simulink model "tesdoang"  (R2024a)
settings: Solver=FixedStepAuto  StartTime=0.0  StopTime=10  FixedStep=1e-5  RelTol=1e-3
values from neighbouring files (symbols this model uses):
  C_inv = (r*(Pinv/3)*al*(-be+al-1))/(100*Vac_l_rms*Vin_inv*wn*(al-be))    [main_v2gg2v.m]    (also in script.m = 0.00198943678865)
  C_mppt = 20*(Iout_mppt*D_mppt)/(deltaV*fs_mppt)    (= 0.0948148148148)    [main_v2gg2v.m]    (also in script.m)
  cap_bat = 2000    [main_v2gg2v.m]    (also in script.m)
  Cbat_buck = deltaI_bat/(8*fs_bat*deltaV_bat)    (= 0.00133333333333)    [main_v2gg2v.m]    (also in script.m)
  Cdc = 30e-3    (= 0.03)    [main_v2gg2v.m]    (also in script.m)
  Cdc_boost = 50*Cbat_buck    (= 0.0666666666667)    [main_v2gg2v.m]    (also in script.m)
  D_g1 = 5    [script.m]
  D_g2 = 5    [script.m]
  Elf_g1 = 1.06    [script.m]
  Elf_g2 = 1.15    [script.m]
  fg = 50    [main_v2gg2v.m]    (also in script.m)
  H_g1 = 4    [script.m]
  H_g2 = 1.8    [script.m]
  L_bat = (Vbat*(Vdc_link-Vbat))/(deltaI_bat*fs_bat*Vdc_link)    (= 0.001875)    [main_v2gg2v.m]    (also in script.m)
  L_mppt = 1*(Vpv*D_mppt)/(deltaI*fs_mppt)    (= 0.000161333333333)    [main_v2gg2v.m]    (also in script.m)
  Lmin_inv = (100*Vac_l_rms*Vin_inv*(al-be))/(wn*r*(Pinv/3)*(-be+al-1))    [main_v2gg2v.m]    (also in script.m = 0.000611154981473)
  pairPoles_g1 = 2    [script.m]
  pairPoles_g2 = 3    [script.m]
  Pinv = 2e6    (= 2000000)    [main_v2gg2v.m]    (also in script.m)
  Pmlf_g1 = 0.84    [script.m]
  Pmlf_g2 = 0.82    [script.m]
  R_g1 = 0.015    [script.m]
  R_g2 = 0.02    [script.m]
  Rdroop_g1 = 0.05    [script.m]
  Rdroop_g2 = 0.06    [script.m]
  RL_mppt_dummy = Vdc_link^2/Ppv    (= 1.125)    [main_v2gg2v.m]    (also in script.m)
  Sbase = 1e6    (= 1000000)    [main_v2gg2v.m]    (also in script.m)
  Snom_g1 = 7e6    (= 7000000)    [script.m]
  Snom_g2 = 5e6    (= 5000000)    [script.m]
  Tg_g1 = 0.4    [script.m]
  Tg_g2 = 0.25    [script.m]
  Vac_grid = Vbase    (= 345000)    [script.m]
  Vac_inv = 800    [main_v2gg2v.m]    (also in script.m)
  Vbat = 750    [main_v2gg2v.m]    (also in script.m)
  X_g1 = 0.3    [script.m]
  X_g2 = 0.35    [script.m]
  Xline_12 = 7/6    (= 1.16666666667)    [script.m]
  Xline_13 = 8/6    (= 1.33333333333)    [script.m]
  Xline_23 = 4/6    (= 0.666666666667)    [script.m]
  Zbase = Vbase^2/Sbase    (= 119025)    [main_v2gg2v.m]    (also in script.m)
undefined symbols (not defined in the file or in its folder): A, Acid, B, C, D1, Delta, DiscIntNeverNeededParam, K_lqr, L_kal, Lead
libraries: spsGroundLib x14, eeGeneralControl x10, spsSeriesRLCBranchLib x9, simulink x7, spsThreePhaseVIMeasurementLib x6, slpidlib x6, spsThreePhaseSeriesRLCBranchLib x6, spsCurrentMeasurementLib x5, spsBatteryLib x3, spsVoltageMeasurementLib x3, spsRMSLib x3, spsThreePhaseParallelRLCLoadLib x3
(part 1 of 2)
settings Model: SimulationMode=accelerator  Creator=hp  LastModifiedBy=hp
settings DebuggingCC: AlgebraicLoopMsg=error  ArtificialAlgebraicLoopMsg=error  BlockPriorityViolationMsg=error  SolverPrmCheckMsg=warning  StateNameClashWarn=warning  OperatingPointInterfaceChecksumMismatchMsg=error
settings HardwareCC: ProdHWDeviceType=AMD->x86-64 (Windows64)
settings DiagnosticsConfigSet: SimMechanicsInvalidVisualProperty=error  SimMechanicsCrossSectionNullEdge=error  SimMechanicsUnconnectedFramePorts=error  SimMechanicsUnconnectedGeometryPorts=error  SimMechanicsRedundantBlock=error  SimMechanicsConflictingReferenceFrames=error  SimMechanicsUnsatisfiedHighPriorityTargets=error

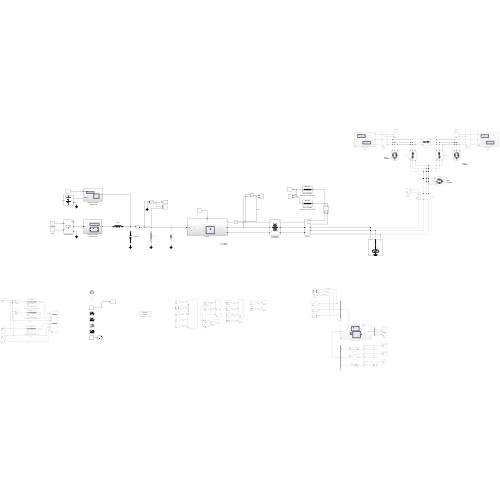
[thumbnail: Simulink's stored preview of the top-level diagram]
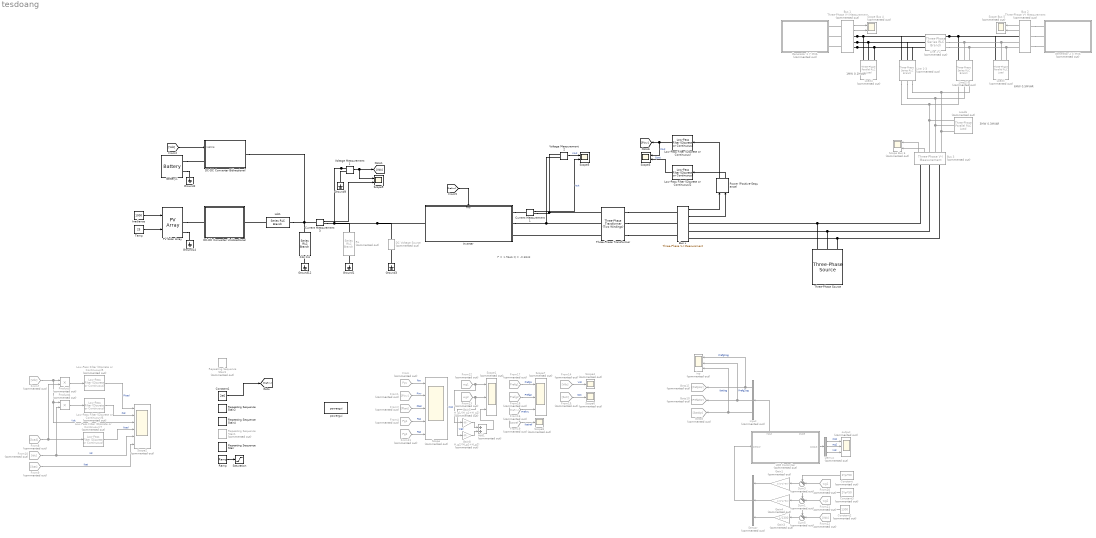
== system tesdoang ==
  note: P = 1.96e6
      | Q = -0.6843
  note: 6MW
      | 0.5MVAR
  note: 3MW
      | 0.3MVAR
  note: 1MW
      | 0.1MVAR
  Add1 : Sum  Commented=on
  Battery1 : spsBatteryLib/Battery  BatType=Lead-Acid  ShowTempParam=off  ThermalPreset="12.8V  40Ah  (LiFeMgPO4)"  ShowAgeParam=off  NomV=Vbat  NomQ=cap_bat  SOC=50  Batt_Tr=2  PresetModel=off  MaxQ=cap_bat  MinV=0.8*Vbat  FullV=1.1*Vbat  Dis_rate=Inom_bat  R=0.002  Normal_OP=0.9*cap_bat  expZone="[780   20]"  current=[250 500 750 1000]  Units=Ampere-hour  Tci=20  NomT=20  T2=-30  MaxQ2=4.8  FullV2=7.1  Normal_OP2=5.655  expZone2="[6.58           1]"  Rca=0.6  ti=2000  Dp=0  Neq0=0  Tsim=1e6  Ta1=25  Qeol=5.4*0.9  Reol=0.013333*1.2  Char_age=[2.3478, 3]  Dis_age=[2.3478, 10]  N1=1500  N2=10500  N3=1000  N4=1400  Ta2=45  N5=950
  Bus 1 : spsThreePhaseVIMeasurementLib/Three-Phase V-I Measurement  Commented=on  VoltageMeasurement=phase-to-phase  SetLabelV=off  LabelV=Vabc  Vpu=off  VpuLL=off  CurrentMeasurement=yes  SetLabelI=off  LabelI=Iabc  Ipu=off  Pbase=100e6  Vbase=13.8e3  OutputType=Complex  PhasorSimulation=off  PSBequivalent=0
  Bus 2 : spsThreePhaseVIMeasurementLib/Three-Phase V-I Measurement  Commented=on  VoltageMeasurement=phase-to-phase  SetLabelV=off  LabelV=Vabc  Vpu=off  VpuLL=off  CurrentMeasurement=yes  SetLabelI=off  LabelI=Iabc  Ipu=off  Pbase=100e6  Vbase=13.8e3  OutputType=Complex  PhasorSimulation=off  PSBequivalent=0
  Bus 3 : spsThreePhaseVIMeasurementLib/Three-Phase V-I Measurement  Commented=on  VoltageMeasurement=phase-to-phase  SetLabelV=off  LabelV=Vabc  Vpu=off  VpuLL=off  CurrentMeasurement=yes  SetLabelI=off  LabelI=Iabc  Ipu=off  Pbase=100e6  Vbase=13.8e3  OutputType=Complex  PhasorSimulation=off  PSBequivalent=0
  Bus x : spsThreePhaseVIMeasurementLib/Three-Phase V-I Measurement  VoltageMeasurement=phase-to-ground  SetLabelV=off  LabelV=Vabc  Vpu=off  VpuLL=off  CurrentMeasurement=yes  SetLabelI=off  LabelI=Iabc  Ipu=off  Pbase=100e6  Vbase=13.8e3  OutputType=Complex  PhasorSimulation=off  PSBequivalent=0
  Cdc link : spsSeriesRLCBranchLib/Series RLC Branch  LConnTagsString=__new0  RConnTagsString=__new0  BranchType=C  Resistance=0.001  Inductance=1e-3  SetiL0=off  InitialCurrent=0  Capacitance=Cdc  Setx0=on  InitialVoltage=1500  Measurements=None
  Constant : Constant  Commented=on  Value=2*pi*50  SampleTime=1e-6
  Constant1 : Constant  Value=2e6  SampleTime=1e-5
  Constant2 : Constant  Commented=on  Value=1300  SampleTime=1e-6
  Constant3 : Constant  Commented=on  Value=2*pi*50  SampleTime=1e-6
  Current Measurement1 : spsCurrentMeasurementLib/Current Measurement  PhasorSimulation=off  OutputType=Complex  PSBequivalent=0
  Current Measurement3 : spsCurrentMeasurementLib/Current Measurement  PhasorSimulation=off  OutputType=Complex  PSBequivalent=0
  DC Voltage Source : spsDCVoltageSourceLib/DC Voltage Source  Commented=on  Amplitude=1500  Measurements=None
  DC-DC Converter Bidirectional : Subsystem
  DC-DC Converter Unidirectional : Subsystem
  Demux : Demux  Commented=on  Outputs=3
  From : From  Commented=on  GotoTag=Ppv  TagVisibility=global
  From1 : From  Commented=on  GotoTag=Pinv
  From10 : From  Commented=on  GotoTag=idc
  From11 : From  Commented=on  GotoTag=Pg2  TagVisibility=global
  From12 : From  Commented=on  GotoTag=wg1  TagVisibility=global
  From13 : From  Commented=on  GotoTag=wg2  TagVisibility=global
  From14 : From  Commented=on  GotoTag=Vdc
  From15 : From  Commented=on  GotoTag=SoC
  From16 : From  Commented=on  GotoTag=Prefinv
  From17 : From  Commented=on  GotoTag=Prefg1  TagVisibility=global
  From18 : From  Commented=on  GotoTag=Prefg2  TagVisibility=global
  From19 : From  Commented=on  GotoTag=ibatref  TagVisibility=global
  From20 : From  Commented=on  GotoTag=wg1  TagVisibility=global
  From21 : From  Commented=on  GotoTag=wg2  TagVisibility=global
  From22 : From  Commented=on  GotoTag=Vdc
  From3 : From  Commented=on  GotoTag=Pbat
  From4 : From  Commented=on  GotoTag=Pg1  TagVisibility=global
  From7 : From  Commented=on  GotoTag=Vdc
  From8 : From  Commented=on  GotoTag=iload
  From9 : From  Commented=on  GotoTag=ibat
  Gain1 : Gain  Commented=on  Gain=1/(2*pi*50)
  Gain3 : Gain  Commented=on  Gain=1/1300
  Gain4 : Gain  Commented=on  Gain=1/(2*pi*50)
  Gain5 : Gain  Commented=on  Gain=H_g1/(H_g1+H_g2)
  Gain8 : Gain  Commented=on  Gain=H_g2/(H_g1+H_g2)
  Generator 1 7 MVA : Subsystem  Commented=on
  Generator 2 5 MVA : Subsystem  Commented=on
  Goto10 : Goto  Commented=on  GotoTag=Prefg2lqr
  Goto11 : Goto  Commented=on  GotoTag=Prefg1lqr
  Goto8 : Goto  Commented=on  GotoTag=ibatlqr
  Ground{1..3,9,12,14} (6 alike) : spsGroundLib/Ground  LConnTagsString=a
  Inverter : Subsystem
      settings: PortSchema="{\"entries\":[{\"content\":{\"sides\":[{\"content\":{\"connectorIds\":[\"LConn1\"]},\"type\":\"ConnectorPlacement.EquallySpacedRectSide\",\"uuid\":\"d809accf-09b8-4494-81bc-1d69e3e04452\"},{\"content\":{\"connectorIds\":[\"RConn1\",\"RConn2\",\"RConn3\"],\"side\":\"RIGHT\"},\"type\":\"ConnectorPlacement.EquallySpacedRectSide\",\"uuid\":\"7565151a-cc1d-4af3-8273-276aca7ed7db\"},{\"content\":{\"connectorIds\":[\"In1\"],\"side\":\"TOP\"},\"type\":\"ConnectorPlacement.EquallySpacedRectSide\",\"uuid\":\"f5878d9b-03b5-4d14-a112-3c604c7d3945\"}]},\"type\":\"ConnectorPlacement.EquallySpacedConnector\",\"uuid\":\"541ee9b8-5fee-4c0b-9c3d-f387ea2048a9\"}],\"packageUris\":[\"http://schema.mathworks.com/mf0/Connector/R2020b\"],\"version\":\"1.0\"}"
  Irradiance : Constant  Value=1000
  LQG Controller : Subsystem  Commented=on
      settings: PortSchema="{\"entries\":[{\"content\":{\"sides\":[{\"content\":{\"connectorIds\":[\"In1\"]},\"type\":\"ConnectorPlacement.EquallySpacedRectSide\",\"uuid\":\"67e13ba4-2390-40ae-81bd-722c33c9b0aa\"},{\"content\":{\"connectorIds\":[\"Out1\"],\"side\":\"RIGHT\"},\"type\":\"ConnectorPlacement.EquallySpacedRectSide\",\"uuid\":\"10755834-48e2-4eb7-99fd-7f61b1a0bfbb\"},{\"content\":{\"connectorIds\":[\"Out2\",\"Out3\"],\"side\":\"TOP\"},\"type\":\"ConnectorPlacement.EquallySpacedRectSide\",\"uuid\":\"f960e436-fda3-4bd6-9c33-52dbb73af01f\"},{\"content\":{\"side\":\"BOTTOM\"},\"type\":\"ConnectorPlacement.EquallySpacedRectSide\",\"uuid\":\"368e05d1-fe46-44bb-9933-6722abe24781\"}]},\"type\":\"ConnectorPlacement.EquallySpacedConnector\",\"uuid\":\"2a48d2f2-f765-4588-a7ff-7a9f3a9a840b\"}],\"packageUris\":[\"http://schema.mathworks.com/mf0/Connector/R2020b\"],\"version\":\"1.0\"}"
  Ldc1 : spsSeriesRLCBranchLib/Series RLC Branch  LConnTagsString=__new0  RConnTagsString=__new0  BranchType=L  Resistance=0.002  Inductance=10e-3  SetiL0=off  InitialCurrent=0  Capacitance=5e-3  Setx0=on  InitialVoltage=0  Measurements=None
  Line 1-2 : spsThreePhaseSeriesRLCBranchLib/Three-Phase Series RLC Branch  Commented=on  LConnTagsString=A|B|C  RConnTagsString=A|B|C  BranchType=RL  Resistance=50*(Xline_12*Zbase)/(2*pi*fg)  Inductance=(Xline_12*Zbase)/(2*pi*fg)  Capacitance=1e-6  Measurements=None
  Line 1-3 : spsThreePhaseSeriesRLCBranchLib/Three-Phase Series RLC Branch  Commented=on  LConnTagsString=A|B|C  RConnTagsString=A|B|C  BranchType=RL  Resistance=50*(Xline_13*Zbase)/(2*pi*fg)  Inductance=(Xline_13*Zbase)/(2*pi*fg)  Capacitance=1e-6  Measurements=None
  Line 2-3 : spsThreePhaseSeriesRLCBranchLib/Three-Phase Series RLC Branch  Commented=on  LConnTagsString=A|B|C  RConnTagsString=A|B|C  BranchType=RL  Resistance=50*(Xline_23*Zbase)/(2*pi*fg)  Inductance=(Xline_23*Zbase)/(2*pi*fg)  Capacitance=1e-6  Measurements=None
  Load4 : spsThreePhaseParallelRLCLoadLib/Three-Phase Parallel RLC Load  Commented=on  LConnTagsString=A|B|C  Configuration=Y (grounded)  NominalVoltage=(230000)*1  Vabc=[1e3 1e3 1e3]  Vabcp=[1e3 1e3 1e3]  NominalFrequency=50  UnbalancedPower=off  ActivePower=1000000  InductivePower=100000  CapacitivePower=0  Pabc=[10e3 9e3 11e3]  QLabc=[100 90 110]  QCabc=[100 90 110]  Pabcp=[10e3 9e3 11e3]  QLabcp=[100 90 110]  QCabcp=[100 90 110]  Measurements=None  LoadType=constant PQ
  Load5 : spsThreePhaseParallelRLCLoadLib/Three-Phase Parallel RLC Load  Commented=on  LConnTagsString=A|B|C  Configuration=Y (grounded)  NominalVoltage=(230000)*1  Vabc=[1e3 1e3 1e3]  Vabcp=[1e3 1e3 1e3]  NominalFrequency=50  UnbalancedPower=off  ActivePower=6000000  InductivePower=500000  CapacitivePower=0  Pabc=[10e3 9e3 11e3]  QLabc=[100 90 110]  QCabc=[100 90 110]  Pabcp=[10e3 9e3 11e3]  QLabcp=[100 90 110]  QCabcp=[100 90 110]  Measurements=None  LoadType=constant PQ
  Load6 : spsThreePhaseParallelRLCLoadLib/Three-Phase Parallel RLC Load  Commented=on  LConnTagsString=A|B|C  Configuration=Y (grounded)  NominalVoltage=230e3  Vabc=[1e3 1e3 1e3]  Vabcp=[1e3 1e3 1e3]  NominalFrequency=50  UnbalancedPower=off  ActivePower=3000000  InductivePower=300000  CapacitivePower=0  Pabc=[10e3 9e3 11e3]  QLabc=[100 90 110]  QCabc=[100 90 110]  Pabcp=[10e3 9e3 11e3]  QLabcp=[100 90 110]  QCabcp=[100 90 110]  Measurements=None  LoadType=constant PQ
  Low-Pass Filter (Discrete or Continuous) : eeGeneralControl/Low-Pass Filter (Discrete or Continuous)  K=1  T=1/(2*pi*5)  B=inf  A=-inf  init_option=Inherited from block input  x0=0  Ts=-1
  Low-Pass Filter (Discrete or Continuous)2 : eeGeneralControl/Low-Pass Filter (Discrete or Continuous)  K=1  T=1/(2*pi*5)  B=inf  A=-inf  init_option=Inherited from block input  x0=0  Ts=-1
  Low-Pass Filter (Discrete or Continuous)5 : eeGeneralControl/Low-Pass Filter (Discrete or Continuous)  Commented=on  K=1  T=1/(2*pi*50)  B=inf  A=-inf  init_option=Inherited from block input  x0=0  Ts=-1
  Low-Pass Filter (Discrete or Continuous)6 : eeGeneralControl/Low-Pass Filter (Discrete or Continuous)  Commented=on  K=1  T=1/(2*pi*50)  B=inf  A=-inf  init_option=Inherited from block input  x0=0  Ts=-1
  Low-Pass Filter (Discrete or Continuous)7 : eeGeneralControl/Low-Pass Filter (Discrete or Continuous)  Commented=on  K=1  T=1/(2*pi*50)  B=inf  A=-inf  init_option=Inherited from block input  x0=0  Ts=-1
  PV Solar Array : spsPVArrayLib/PV Array  Npar=278  Nser=15  PlotType=array @ 1000 W/m2 & specified temperatures  S_vec=[ 1000 800 500 300 100 ]  Temp_C_vec=[ 20 25 30 35 ]  ModuleName=Sunpower SPR-X22-480-COM  PlotWhenSelected=off  Pm=480.32  Ncell=128  Voc=92.9  Isc=6.48  Vm=79  Im=6.08  beta_Voc_pc=-0.293  alpha_Isc_pc=0.031003  beta_Voc=-0.2722  alpha_Isc=0.002009  IL=6.4884  I0=1.5908e-11  nI=1.0576  Rsh=598.2816  Rs=0.48607  RobustModel=off  RobustCellTemperature=313.3991  BAL=on  Tc=1e-6  Tfilter=5e-5
  Power (Positive-Sequence) : spsPowerPositiveSequenceLib/Power (Positive-Sequence)  Freq=50  Vinit=[0, 0]  Iinit=[0, 0]  Ts=1e-5
      settings: LibrarySourceBlock=|
      | sps_lib/Sensors and Measurements/Power
      | (Positive-Sequence)
  Product3 : Product  Commented=on
  Product4 : Product  Commented=on
  RL : spsSeriesRLCBranchLib/Series RLC Branch  Commented=on  LConnTagsString=__new0  RConnTagsString=__new0  BranchType=R  Resistance=RL_mppt_dummy  Inductance=1e-3  SetiL0=off  InitialCurrent=0  Capacitance=30e-3  Setx0=on  InitialVoltage=1300  Measurements=None
  Ramp : simulink/Sources/Ramp  slope=0.5e6  start=1  InitialOutput=0
  Repeating Sequence Stair : simulink/Sources/Repeating Sequence Stair  OutValues=[0 0 0 0 0.1e6 0.2e6 0.3e6 0.4e6 0.5e6 0.6e6 0.7e6 0.8e6 0.9e6 1.0e6 0.5e6 0.1e6 0.05e6 0.025e6 0.0125e6 1e6].'  tsamp=0.5  OutMin=[]  OutMax=[]  OutDataTypeStr=double  OutputDataTypeScalingMode=double  OutDataType=fixdt(0,8)  ConRadixGroup=Best Precision: Vector-wise  OutScaling=2^-12
  Repeating Sequence Stair1 : simulink/Sources/Repeating Sequence Stair  Commented=on  OutValues=[0 0 0 0 1e6 0 1e6 0].'  tsamp=0.5  OutMin=[]  OutMax=[]  OutDataTypeStr=double  OutputDataTypeScalingMode=double  OutDataType=fixdt(0,8)  ConRadixGroup=Best Precision: Vector-wise  OutScaling=2^-12
  Repeating Sequence Stair2 : simulink/Sources/Repeating Sequence Stair  OutValues=[0.3e6 0.3e6 0.2e6 0.5e6 0.4e6 0.7e6 0.5e6 0.9e6 1e6 0.5e6 0.1e6 0.5e6].'  tsamp=1  OutMin=[]  OutMax=[]  OutDataTypeStr=double  OutputDataTypeScalingMode=double  OutDataType=fixdt(0,8)  ConRadixGroup=Best Precision: Vector-wise  OutScaling=2^-12
  Repeating Sequence Stair3 : simulink/Sources/Repeating Sequence Stair  Commented=on  OutValues=[0 0.3e6 0.6e6 0.8e6 0.9e6 1e6 0.9e6 0.8e6 0.6e6 0.3e6].'  tsamp=1  OutMin=[]  OutMax=[]  OutDataTypeStr=double  OutputDataTypeScalingMode=double  OutDataType=fixdt(0,8)  ConRadixGroup=Best Precision: Vector-wise  OutScaling=2^-12
  Repeating Sequence Stair4 : simulink/Sources/Repeating Sequence Stair  OutValues=[0 0 0.5e6 1e6 1e6 0.5e6 0.1e6 ].'  tsamp=1  OutMin=[]  OutMax=[]  OutDataTypeStr=double  OutputDataTypeScalingMode=double  OutDataType=fixdt(0,8)  ConRadixGroup=Best Precision: Vector-wise  OutScaling=2^-12
  Saturation : Saturate  UpperLimit=2e6  LowerLimit=0
  Scope : Scope  Commented=on  NumInputPorts=5
  Scope Bus 4 : Scope  Commented=on  NumInputPorts=2
  Scope Bus 5 : Scope  Commented=on  NumInputPorts=2
  Scope Bus 6 : Scope  Commented=on  NumInputPorts=2
  Scope1 : Scope  Commented=on  NumInputPorts=3
  Scope2 : Scope  Commented=on  NumInputPorts=6
  Scope3 : Scope  NumInputPorts=2
  Scope4 : Scope  Commented=on
  Scope5 : Scope  NumInputPorts=2
  Scope6 : Scope  Commented=on
  Scope7 : Scope  Commented=on  NumInputPorts=3
  Scope8 : Scope  Commented=on
  Scope9 : Scope  NumInputPorts=2
  Sensor : Mux  Commented=on  Inputs=3
  Sum1 : Sum  Commented=on  Inputs=-+|
  Sum3 : Sum  Commented=on  Inputs=-+|
  Sum5 : Sum  Commented=on  Inputs=-+|
  Temp : Constant  Value=25
  Three-Phase Transformer : spsThreePhaseTransformerTwoWindingsLib/Three-Phase Transformer (Two Windings)  Winding1Connection=Yg  Winding2Connection=Delta (D1)  CoreType=Three single-phase transformers  SetSaturation=off  Hysteresis=off  DataFile='hysteresis'  SetInitialFlux=off  Measurements=None  UNITS=pu  NominalPower=[ Pinv*2 , fg ]  Winding1=[Vac_grid 1e-6 1e-6]  Winding2=[Vac_inv 1e-6 1e-6]  Rm=500  Lm=1000  L0=0.5  Saturation=[0 0;0.01 0.9;0.05 1]  InitialFluxes=[-1.0025142026259 0.501432695325379 0.501081507300505]  BreakLoop=off  DiscreteSolver=Trapezoidal iterative  DataType=off  TransfoNumber=1
  Three-Phase Source : spsThreePhaseSourceLib/Three-Phase Source  InternalConnection=Yg  VoltagePhases=off  Voltage=Vac_grid  PhaseAngle=0  Voltage_phases=[25e3 25e3 25e3]/sqrt(3)  PhaseAngles_phases=[0 -120 +120]  Frequency=fg  NonIdealSource=off  SpecifyImpedance=off  Resistance=0.8929  Inductance=16.58e-3  ShortCircuitLevel=100e6  BaseVoltage=25e3  XRratio=7  BusType=swing  Pref=10e3  Qref=0  Prefabc=[10e3, 10e3, 10e3]  Qrefabc=[0, 0, 0]  Qmin=-inf  Qmax=inf
  Voltage Measurement1 : spsVoltageMeasurementLib/Voltage Measurement  PhasorSimulation=off  OutputType=Complex  PSBequivalent=0
  Voltage Measurement2 : spsVoltageMeasurementLib/Voltage Measurement  PhasorSimulation=off  OutputType=Complex  PSBequivalent=0
  inp : Scope  Commented=on  NumInputPorts=3
  input : Demux  Commented=on  Outputs=3
  output : Scope  Commented=on  NumInputPorts=3
  powergui : spspowerguiLib/powergui  Priority=1  SimulationMode=Discrete  SampleTime=1e-5  frequency=60  Iterations=200  frequencyindice=0  Pbase=100e6  ErrMax=1e-4  UnitsV=kV  UnitsW=MW  buscounter=0  FunctionMessages=off  echomessages=off  EnableUseOfTLC=on  CurrentSourceSwitches=off  DisableSnubberDevices=off  DisableRonSwitches=off  DisableVfSwitches=off  DisplayEquations=off  AutomaticDiscreteSolvers=off  SolverType=Tustin/Backward Euler (TBE)  Interpol=off  ExternalGateDelay=off  methode=off  Ts=100  x0status=blocks  SPID=on  SwTol=0  HookPort=off  NonlinearTolerance=1e-4  nMaxIteration=100  ContinueOnMaxIteration=off  RestoreLinks=warning  ResistiveCurrentMeasurement=off  Frange=[0:2:500]  Ylog=off  Xlog=on  ShowGrid=off  save=off  variable=ZData  structure=0  ZoomFFT=off  StartTime=0.0  cycles=1  DisplayStyle=1  fundamental=60  FreqAxis=off  MaxFrequency=1000  frequencyindicesteady=1  RmsSteady=1  display=off
  wires:
  Bus 1/2 -> Scope Bus 4/2
  Bus 2/2 -> Scope Bus 5/2
  Bus 3/2 -> Scope Bus 6/2
  Bus 1/1 -> Scope Bus 4/1
  Bus 2/1 -> Scope Bus 5/1
  Ramp/1 -> Saturation/1
  Constant1/1 -> [Prefinv]
  Bus 3/1 -> Scope Bus 6/1
  Power (Positive-Sequence)/2 -> Low-Pass Filter (Discrete or Continuous)2/1
  Power (Positive-Sequence)/1 -> Low-Pass Filter (Discrete or Continuous)/1
  Bus x/1 -> Power (Positive-Sequence)/1
  Bus x/2 -> Power (Positive-Sequence)/2
  Low-Pass Filter (Discrete or Continuous)/1 -> [Pinv], Scope3/1  "Pout"
  Low-Pass Filter (Discrete or Continuous)2/1 -> Scope3/2  "Qout"
  Temp/1 -> PV Solar Array/2
  Irradiance/1 -> PV Solar Array/1
  [Vdc] -> DC-DC Converter Bidirectional/1(Vdclink)
  From10/1 -> Product4/2, Scope2/5  "idc"
  Product3/1 -> Low-Pass Filter (Discrete or Continuous)5/1
  Low-Pass Filter (Discrete or Continuous)6/1 -> Scope2/2  "Pdc"
  From8/1 -> Product3/2, Low-Pass Filter (Discrete or Continuous)7/1
  Low-Pass Filter (Discrete or Continuous)5/1 -> Scope2/1  "Pload"
  From9/1 -> Scope2/6  "ibat"
  From7/1 -> Scope2/3, Product4/1, Product3/1  "Vdc"
  Product4/1 -> Low-Pass Filter (Discrete or Continuous)6/1
  Low-Pass Filter (Discrete or Continuous)7/1 -> Scope2/4  "iload"
  From12/1 -> Gain5/1, Scope1/1  "wg1"
  From13/1 -> Gain8/1, Scope1/2  "wg2"
  From15/1 -> Scope6/1  "SoC"
  From14/1 -> Scope4/1  "Vdc"
  From/1 -> Scope/1  "Ppv"
  From1/1 -> Scope/2  "Pinv"
  From3/1 -> Scope/3  "Pbat"
  From4/1 -> Scope/4  "Pg1"
  From11/1 -> Scope/5  "Pg2"
  From17/1 -> Scope7/1  "Prefg1"
  From18/1 -> Scope7/2  "Prefg2"
  From16/1 -> Scope7/3  "Prefinv"
  From19/1 -> Scope8/1  "ibatref"
  Constant/1 -> Sum3/1
  Gain1/1 -> Sensor/1
  Sum3/1 -> Gain1/1
  Sum5/1 -> Gain3/1
  Gain3/1 -> Sensor/3
  From22/1 -> Sum5/2
  Constant2/1 -> Sum5/1
  input/1 -> Goto11/1, inp/1  "Prefg1lqg"
  input/2 -> Goto10/1, inp/2  "Prefg2lqg"
  input/3 -> Goto8/1, inp/3  "ibatlqg"
  Demux/1 -> output/1  "wg1"
  Demux/2 -> output/2  "wg2"
  [Prefinv] -> Inverter/1(Pref)
  Sensor/1 -> LQG Controller/1(sensor)
  LQG Controller/2(input) -> input/1
  LQG Controller/1(output) -> Demux/1
  Demux/3 -> output/3  "Vdc"
  Sum1/1 -> Gain4/1
  Gain4/1 -> Sensor/2
  Constant3/1 -> Sum1/1
  From20/1 -> Sum3/2
  From21/1 -> Sum1/2
  Gain8/1 -> Add1/2
  Gain5/1 -> Add1/1
  Add1/1 -> Scope1/3
  Voltage Measurement1/1 -> [Vdc], Scope9/1
  Current Measurement3/1 -> Scope9/2
  Voltage Measurement2/1 -> Scope5/1  "Vout"
  Current Measurement1/1 -> Scope5/2  "iout"
  connections:
  Line 1-2/RConn1 -- Line 2-3/RConn1 -- Load5/LConn1 -- Bus 2/RConn1
  Load5/LConn2 -- Bus 2/RConn2 -- Line 2-3/RConn2 -- Line 1-2/RConn2
  Line 2-3/LConn2 -- Load6/LConn2 -- Bus 3/RConn2 -- Line 1-3/RConn2
  Line 2-3/LConn1 -- Load6/LConn1 -- Bus 3/RConn1 -- Line 1-3/RConn1
  Bus 1/RConn1 -- Load4/LConn1 -- Line 1-3/LConn1 -- Line 1-2/LConn1
  Bus 1/RConn2 -- Load4/LConn2 -- Line 1-3/LConn2 -- Line 1-2/LConn2
  Line 2-3/LConn3 -- Load6/LConn3 -- Bus 3/RConn3 -- Line 1-3/RConn3
  Bus 1/RConn3 -- Load4/LConn3 -- Line 1-3/LConn3 -- Line 1-2/LConn3
  Load5/LConn3 -- Bus 2/RConn3 -- Line 2-3/RConn3 -- Line 1-2/RConn3
  Bus 1/LConn3 -- Generator 1 7 MVA/RConn3
  Bus 2/LConn1 -- Generator 2 5 MVA/RConn1
  Bus 1/LConn1 -- Generator 1 7 MVA/RConn1
  Bus 2/LConn3 -- Generator 2 5 MVA/RConn3
  Bus 1/LConn2 -- Generator 1 7 MVA/RConn2
  Bus 2/LConn2 -- Generator 2 5 MVA/RConn2
  Current Measurement1/RConn1 -- Three-Phase Transformer/RConn1 -- Voltage Measurement2/LConn1
  PV Solar Array/RConn1 -- DC-DC Converter Unidirectional/LConn1
  Ldc1/LConn1 -- DC-DC Converter Unidirectional/RConn1
  Ground12/LConn1 -- Cdc link/RConn1
  PV Solar Array/RConn2 -- Ground14/LConn1
  Voltage Measurement1/LConn2 -- Ground9/LConn1
  Inverter/RConn2 -- Three-Phase Transformer/RConn2 -- Voltage Measurement2/LConn2
  Inverter/RConn1 -- Current Measurement1/LConn1
  Cdc link/LConn1 -- DC-DC Converter Bidirectional/RConn1 -- Ldc1/RConn1 -- Current Measurement3/LConn1
  Battery1/LConn2 -- Ground2/LConn1
  Battery1/LConn1 -- DC-DC Converter Bidirectional/LConn1
  Ground1/LConn1 -- RL/RConn1
  Ground3/LConn1 -- DC Voltage Source/LConn1
  Three-Phase Source/RConn3 -- Bus 3/LConn3 -- Bus x/RConn3
  Three-Phase Source/RConn2 -- Bus 3/LConn2 -- Bus x/RConn2
  Three-Phase Source/RConn1 -- Bus 3/LConn1 -- Bus x/RConn1
  Voltage Measurement1/LConn1 -- RL/LConn1 -- DC Voltage Source/RConn1 -- Inverter/LConn1 -- Current Measurement3/RConn1
  Three-Phase Transformer/LConn3 -- Bus x/LConn3
  Three-Phase Transformer/LConn1 -- Bus x/LConn1
  Three-Phase Transformer/LConn2 -- Bus x/LConn2
  Three-Phase Transformer/RConn3 -- Inverter/RConn3

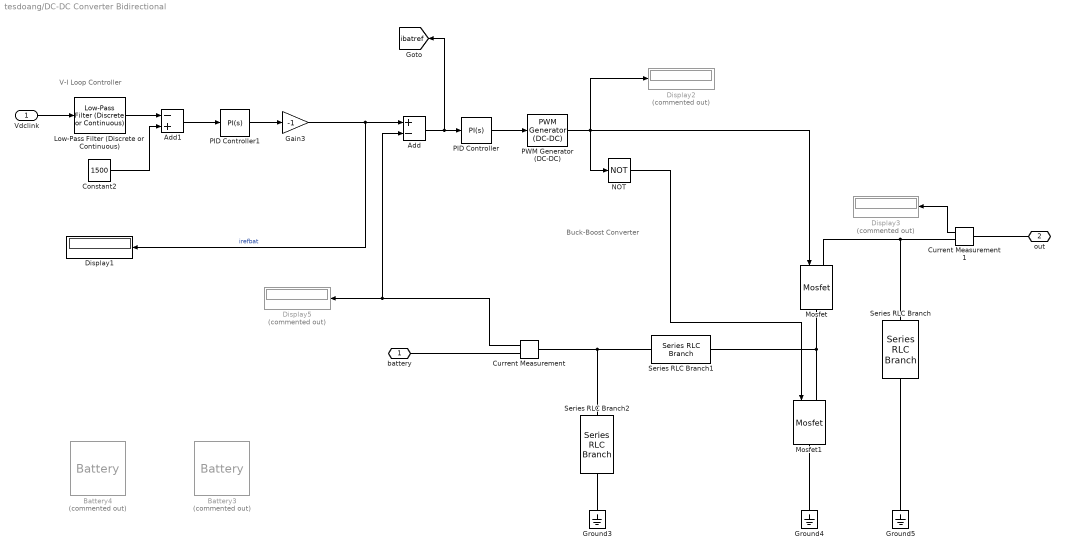
== system tesdoang/DC-DC Converter Bidirectional ==
  note: V-I Loop Controller
  note: Buck-Boost Converter
  Vdclink : Inport
  Add : Sum  Inputs=+-
  Add1 : Sum  Inputs=-+
  Battery3 : spsBatteryLib/Battery  Commented=on  BatType=Lead-Acid  ShowTempParam=off  ThermalPreset="12.8V  40Ah  (LiFeMgPO4)"  ShowAgeParam=off  NomV=Vbat  NomQ=cap_bat  SOC=50  Batt_Tr=30  PresetModel=on  MaxQ=2083.3333  MinV=562.5  FullV=816.6118  Dis_rate=400  R=0.00375  Normal_OP=620.5556  expZone="[763.5691      6.666667]"  current=[250 500 750 1000]  Units=Time  Tci=20  NomT=20  T2=-30  MaxQ2=4.8  FullV2=7.1  Normal_OP2=5.655  expZone2="[6.58           1]"  Rca=0.6  ti=2000  Dp=0  Neq0=0  Tsim=1e6  Ta1=25  Qeol=5.4*0.9  Reol=0.013333*1.2  Char_age=[2.3478, 3]  Dis_age=[2.3478, 10]  N1=1500  N2=10500  N3=1000  N4=1400  Ta2=45  N5=950
  Battery4 : spsBatteryLib/Battery  Commented=on  BatType=Lead-Acid  ShowTempParam=off  ThermalPreset="12.8V  40Ah  (LiFeMgPO4)"  ShowAgeParam=off  NomV=Vbat  NomQ=cap_bat  SOC=50  Batt_Tr=30  PresetModel=off  MaxQ=1000  MinV=0.8*Vbat  FullV=1.1*Vbat  Dis_rate=Inom_bat  R=0.002  Normal_OP=0.9*cap_bat  expZone="[680   10]"  current=[250 500 750 1000]  Units=Time  Tci=20  NomT=20  T2=-30  MaxQ2=4.8  FullV2=7.1  Normal_OP2=5.655  expZone2="[6.58           1]"  Rca=0.6  ti=2000  Dp=0  Neq0=0  Tsim=1e6  Ta1=25  Qeol=5.4*0.9  Reol=0.013333*1.2  Char_age=[2.3478, 3]  Dis_age=[2.3478, 10]  N1=1500  N2=10500  N3=1000  N4=1400  Ta2=45  N5=950
  Constant2 : Constant  Value=1500  SampleTime=1e-5
  Current Measurement : spsCurrentMeasurementLib/Current Measurement  PhasorSimulation=off  OutputType=Complex  PSBequivalent=0
  Current Measurement1 : spsCurrentMeasurementLib/Current Measurement  PhasorSimulation=off  OutputType=Complex  PSBequivalent=0
  Display1 : Display
  Display2 : Display  Commented=on
  Display3 : Display  Commented=on
  Display5 : Display  Commented=on
  Gain3 : Gain  Gain=-1
  Ground3 : spsGroundLib/Ground  LConnTagsString=a
  Ground4 : spsGroundLib/Ground  LConnTagsString=a
  Ground5 : spsGroundLib/Ground  LConnTagsString=a
  Low-Pass Filter (Discrete or Continuous) : eeGeneralControl/Low-Pass Filter (Discrete or Continuous)  K=1  T=1/(2*pi*30)  B=inf  A=-inf  init_option=Inherited from block input  x0=0  Ts=1e-5
  Mosfet : spsMosfetLib/Mosfet  Ron=0.1  Lon=0  Rd=0.01  Vfd=0  IC=0  Rs=1e5  Cs=inf  Measurements=off
  Mosfet1 : spsMosfetLib/Mosfet  Ron=0.1  Lon=0  Rd=0.01  Vfd=0  IC=0  Rs=1e5  Cs=inf  Measurements=off
  NOT : Logic  Operator=NOT  AllPortsSameDT=off  OutDataTypeStr=boolean
  PID Controller : slpidlib/PID Controller  Controller=PI  Form=Parallel  TimeDomain=Continuous-time  UseExternalTs=off  SampleTime=-1  IntegratorMethod=Forward Euler  FilterMethod=Forward Euler  ControllerParametersSource=internal  P=50  I=2000  UseKiTs=off  D=10  UseExternalDerivativeSource=off  N=100  UseFilter=on  TunerSelectOption=Transfer Function Based (PID Tuner App)  InitialConditionSource=internal  InitialConditionForIntegrator=0  InitialConditionForFilter=0  DifferentiatorICPrevScaledInput=0.05  ExternalReset=none  TrackingMode=off  Kt=1  LimitOutput=on  SatLimitsSource=internal  UpperSaturationLimit=0.95  LowerSaturationLimit=0  LinearizeAsGain=on  AntiWindupMode=clamping  Kb=5000  LimitIntegrator=off  UpperIntegratorSaturationLimit=inf  LowerIntegratorSaturationLimit=-inf  POutMin=[]  POutMax=[]  IOutMin=[]  IOutMax=[]  DOutMin=[]  DOutMax=[]  NOutMin=[]  NOutMax=[]  SumOutMin=[]  SumOutMax=[]  SaturationOutMin=[]  SaturationOutMax=[]  PParamMin=[]  PParamMax=[]  IParamMin=[]  IParamMax=[]  DParamMin=[]  DParamMax=[]  NParamMin=[]  NParamMax=[]  KbParamMin=[]  KbParamMax=[]  KtParamMin=[]  KtParamMax=[]  KbOutMin=[]  KbOutMax=[]  KtOutMin=[]  KtOutMax=[]  IntegratorOutMin=[]  IntegratorOutMax=[]  FilterOutMin=[]  FilterOutMax=[]  SumI1OutMin=[]  SumI1OutMax=[]  SumI2OutMin=[]  SumI2OutMax=[]  SumI3OutMin=[]  SumI3OutMax=[]  SumI4OutMin=[]  SumI4OutMax=[]  SumDOutMin=[]  SumDOutMax=[]  DifferentiatorOutMin=[]  DifferentiatorOutMax=[]  FilterDiffOutCoefMin=[]  FilterDiffOutCoefMax=[]  ReciprocalOutMin=[]  ReciprocalOutMax=[]  SumDenOutMin=[]  SumDenOutMax=[]  SumNumOutMin=[]  SumNumOutMax=[]  DivideOutMin=[]  DivideOutMax=[]  UdiffTsProdOutMin=[]  UdiffTsProdOutMax=[]  NTsProdOutMin=[]  NTsProdOutMax=[]  UintegralTsProdOutMin=[]  UintegralTsProdOutMax=[]  UngainTsProdOutMin=[]  UngainTsProdOutMax=[]  ClampingZeroOutDataTypeStr=Inherit: Inherit via back propagation  ClampingZeroOutMin=[]  ClampingZeroOutMax=[]  FilterDenConstantOutDataTypeStr=Inherit: Inherit via back propagation  FilterDenConstantOutMin=[]  FilterDenConstantOutMax=[]  PCopyOutDataTypeStr=Inherit: Inherit via back propagation  PCopyOutMin=[]  PCopyOutMax=[]  NCopyOutDataTypeStr=Inherit: Inherit via back propagation  NCopyOutMin=[]  NCopyOutMax=[]  IntegratorContinuousStateAttributes=''  IntegratorStateMustResolveToSignalObject=off  IntegratorRTWStateStorageClass=Auto  FilterContinuousStateAttributes=''  FilterStateMustResolveToSignalObject=off  FilterRTWStateStorageClass=Auto  ParallelPVariant=InternalParameters  IdealPVariant=Disabled  IVariant=InternalParameters  DVariant=Disabled  IntegratorVariant=Continuous  SatVariant=Enabled  AWVariant=ContClampingParallel  PCopyVariant=Disabled  TRVariant=Disabled  FdbkBlocksVariant=Forward  IdealPFdbkVariant=Disabled  SatFdbkVariant=Disabled  DerivativeFilterVariant=Disabled  NVariant=Disabled  NCopyVariant=Disabled_SignalSpec  FilterICVariant=Disabled  IntegratorICVariant=InternalICs  ExternalResetVariant=Disabled  TRSumVariant=Passthrough  SumFdbkVariant=Disabled  SumVariant=Sum_PI  TsampFilterVariant=InternalTs  TsampNgainVariant=Passthrough  TsampIntegralVariant=Disabled_SignalSpec  ExternalSaturationOutDataTypeStr=Inherit: Same as second input  DerivativeSourceVariant=Disabled
  PID Controller1 : slpidlib/PID Controller  Controller=PI  Form=Parallel  TimeDomain=Continuous-time  UseExternalTs=off  SampleTime=1e-3  IntegratorMethod=Forward Euler  FilterMethod=Forward Euler  ControllerParametersSource=internal  P=10  I=400  UseKiTs=off  D=10  UseExternalDerivativeSource=off  N=100  UseFilter=on  TunerSelectOption=Transfer Function Based (PID Tuner App)  InitialConditionSource=internal  InitialConditionForIntegrator=0.05  InitialConditionForFilter=0  DifferentiatorICPrevScaledInput=0.05  ExternalReset=none  TrackingMode=off  Kt=1  LimitOutput=on  SatLimitsSource=internal  UpperSaturationLimit=cap_bat*1.5  LowerSaturationLimit=-cap_bat*1.5  LinearizeAsGain=on  AntiWindupMode=back-calculation  Kb=5000  LimitIntegrator=off  UpperIntegratorSaturationLimit=inf  LowerIntegratorSaturationLimit=-inf  POutMin=[]  POutMax=[]  IOutMin=[]  IOutMax=[]  DOutMin=[]  DOutMax=[]  NOutMin=[]  NOutMax=[]  SumOutMin=[]  SumOutMax=[]  SaturationOutMin=[]  SaturationOutMax=[]  PParamMin=[]  PParamMax=[]  IParamMin=[]  IParamMax=[]  DParamMin=[]  DParamMax=[]  NParamMin=[]  NParamMax=[]  KbParamMin=[]  KbParamMax=[]  KtParamMin=[]  KtParamMax=[]  KbOutMin=[]  KbOutMax=[]  KtOutMin=[]  KtOutMax=[]  IntegratorOutMin=[]  IntegratorOutMax=[]  FilterOutMin=[]  FilterOutMax=[]  SumI1OutMin=[]  SumI1OutMax=[]  SumI2OutMin=[]  SumI2OutMax=[]  SumI3OutMin=[]  SumI3OutMax=[]  SumI4OutMin=[]  SumI4OutMax=[]  SumDOutMin=[]  SumDOutMax=[]  DifferentiatorOutMin=[]  DifferentiatorOutMax=[]  FilterDiffOutCoefMin=[]  FilterDiffOutCoefMax=[]  ReciprocalOutMin=[]  ReciprocalOutMax=[]  SumDenOutMin=[]  SumDenOutMax=[]  SumNumOutMin=[]  SumNumOutMax=[]  DivideOutMin=[]  DivideOutMax=[]  UdiffTsProdOutMin=[]  UdiffTsProdOutMax=[]  NTsProdOutMin=[]  NTsProdOutMax=[]  UintegralTsProdOutMin=[]  UintegralTsProdOutMax=[]  UngainTsProdOutMin=[]  UngainTsProdOutMax=[]  ClampingZeroOutDataTypeStr=Inherit: Inherit via back propagation  ClampingZeroOutMin=[]  ClampingZeroOutMax=[]  FilterDenConstantOutDataTypeStr=Inherit: Inherit via back propagation  FilterDenConstantOutMin=[]  FilterDenConstantOutMax=[]  PCopyOutDataTypeStr=Inherit: Inherit via back propagation  PCopyOutMin=[]  PCopyOutMax=[]  NCopyOutDataTypeStr=Inherit: Inherit via back propagation  NCopyOutMin=[]  NCopyOutMax=[]  IntegratorContinuousStateAttributes=''  IntegratorStateMustResolveToSignalObject=off  IntegratorRTWStateStorageClass=Auto  FilterContinuousStateAttributes=''  FilterStateMustResolveToSignalObject=off  FilterRTWStateStorageClass=Auto  ParallelPVariant=InternalParameters  IdealPVariant=Disabled  IVariant=InternalParameters  DVariant=Disabled  IntegratorVariant=Continuous  SatVariant=Enabled  AWVariant=BackCalculation  PCopyVariant=Disabled  TRVariant=Disabled  FdbkBlocksVariant=Forward  IdealPFdbkVariant=Disabled  SatFdbkVariant=Disabled  DerivativeFilterVariant=Disabled  NVariant=Disabled  NCopyVariant=Disabled_SignalSpec  FilterICVariant=Disabled  IntegratorICVariant=InternalICs  ExternalResetVariant=Disabled  TRSumVariant=Passthrough  SumFdbkVariant=Disabled  SumVariant=Sum_PI  TsampFilterVariant=InternalTs  TsampNgainVariant=Passthrough  TsampIntegralVariant=Disabled_SignalSpec  ExternalSaturationOutDataTypeStr=Inherit: Same as second input  DerivativeSourceVariant=Disabled
  PWM Generator (DC-DC) : spsPWMGeneratorDCDCLib/PWM Generator (DC-DC)  Fsw=fs_bat  Ts=0
  Series RLC Branch : spsSeriesRLCBranchLib/Series RLC Branch  LConnTagsString=__new0  RConnTagsString=__new0  BranchType=RC  Resistance=1e-3  Inductance=1e-3  SetiL0=off  InitialCurrent=0  Capacitance=Cdc_boost  Setx0=off  InitialVoltage=1300  Measurements=None
  Series RLC Branch1 : spsSeriesRLCBranchLib/Series RLC Branch  LConnTagsString=__new0  RConnTagsString=__new0  BranchType=RL  Resistance=1e-3  Inductance=L_bat  SetiL0=off  InitialCurrent=0  Capacitance=Cdc_boost  Setx0=off  InitialVoltage=0  Measurements=None
  Series RLC Branch2 : spsSeriesRLCBranchLib/Series RLC Branch  LConnTagsString=__new0  RConnTagsString=__new0  BranchType=RC  Resistance=1e-3  Inductance=1e-3  SetiL0=off  InitialCurrent=0  Capacitance=Cbat_buck  Setx0=off  InitialVoltage=650  Measurements=None
  battery : PMIOPort  Side=Left
  out : PMIOPort  Port=2  Side=Right
  tag scope: ibatref=global
  wires:
  Add/1 -> [ibatref], PID Controller/1
  PID Controller/1 -> PWM Generator (DC-DC)/1
  NOT/1 -> Mosfet1/1
  Current Measurement/1 -> Add/2, Display5/1
  PWM Generator (DC-DC)/1 -> Display2/1, Mosfet/1, NOT/1
  Vdclink/1 -> Low-Pass Filter (Discrete or Continuous)/1
  Low-Pass Filter (Discrete or Continuous)/1 -> Add1/1
  Constant2/1 -> Add1/2
  Add1/1 -> PID Controller1/1
  Gain3/1 -> Display1/1, Add/1  "irefbat"
  Current Measurement1/1 -> Display3/1
  PID Controller1/1 -> Gain3/1
  connections:
  Series RLC Branch1/LConn1 -- Mosfet1/LConn1 -- Mosfet/RConn1
  Series RLC Branch1/RConn1 -- Current Measurement/LConn1 -- Series RLC Branch2/LConn1
  Series RLC Branch/LConn1 -- Current Measurement1/RConn1 -- Mosfet/LConn1
  Current Measurement/RConn1 -- battery/RConn1
  Current Measurement1/LConn1 -- out/RConn1
  Ground3/LConn1 -- Series RLC Branch2/RConn1
  Ground4/LConn1 -- Mosfet1/RConn1
  Ground5/LConn1 -- Series RLC Branch/RConn1

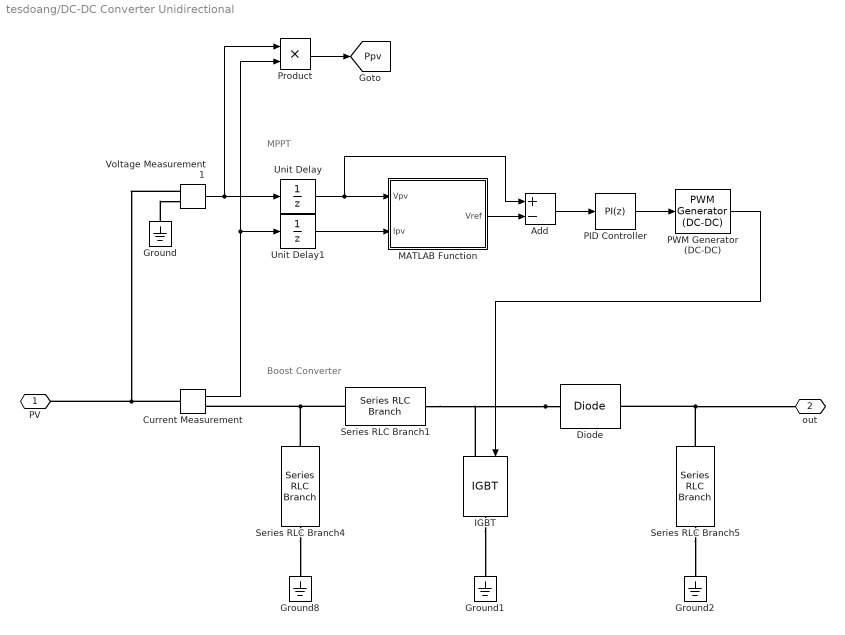
== system tesdoang/DC-DC Converter Unidirectional ==
  note: Boost Converter
  note: MPPT
  Add : Sum  Inputs=+-
  Current Measurement : spsCurrentMeasurementLib/Current Measurement  PhasorSimulation=off  OutputType=Complex  PSBequivalent=0
  Diode : spsDiodeLib/Diode  Ron=0.001  Lon=0  Vf=0.8  IC=0  UseSnubber=0  Rs=500  Cs=250e-9  Measurements=off
  Ground{,1..2,8} (4 alike) : spsGroundLib/Ground  LConnTagsString=a
  IGBT : spsIGBTLib/IGBT  Ron=0.001  Lon=0  Vf=1  Tf=1e-6  Tt=2e-6  IC=0  Rs=1e5  Cs=inf  Measurements=off
  MATLAB Function : MATLAB Function  TreatAsAtomicUnit=on
  PID Controller : slpidlib/PID Controller  Controller=PI  Form=Parallel  TimeDomain=Discrete-time  UseExternalTs=off  SampleTime=-1  IntegratorMethod=Forward Euler  FilterMethod=Forward Euler  ControllerParametersSource=internal  P=0.05  I=500  UseKiTs=off  D=0  UseExternalDerivativeSource=off  N=100  UseFilter=on  TunerSelectOption=Transfer Function Based (PID Tuner App)  InitialConditionSource=internal  InitialConditionForIntegrator=D_mppt  InitialConditionForFilter=0  DifferentiatorICPrevScaledInput=0  ExternalReset=none  TrackingMode=off  Kt=1  LimitOutput=on  SatLimitsSource=internal  UpperSaturationLimit=0.95  LowerSaturationLimit=0.05  LinearizeAsGain=on  AntiWindupMode=clamping  Kb=5  LimitIntegrator=off  UpperIntegratorSaturationLimit=inf  LowerIntegratorSaturationLimit=-inf  POutMin=[]  POutMax=[]  IOutMin=[]  IOutMax=[]  DOutMin=[]  DOutMax=[]  NOutMin=[]  NOutMax=[]  SumOutMin=[]  SumOutMax=[]  SaturationOutMin=[]  SaturationOutMax=[]  PParamMin=[]  PParamMax=[]  IParamMin=[]  IParamMax=[]  DParamMin=[]  DParamMax=[]  NParamMin=[]  NParamMax=[]  KbParamMin=[]  KbParamMax=[]  KtParamMin=[]  KtParamMax=[]  KbOutMin=[]  KbOutMax=[]  KtOutMin=[]  KtOutMax=[]  IntegratorOutMin=[]  IntegratorOutMax=[]  FilterOutMin=[]  FilterOutMax=[]  SumI1OutMin=[]  SumI1OutMax=[]  SumI2OutMin=[]  SumI2OutMax=[]  SumI3OutMin=[]  SumI3OutMax=[]  SumI4OutMin=[]  SumI4OutMax=[]  SumDOutMin=[]  SumDOutMax=[]  DifferentiatorOutMin=[]  DifferentiatorOutMax=[]  FilterDiffOutCoefMin=[]  FilterDiffOutCoefMax=[]  ReciprocalOutMin=[]  ReciprocalOutMax=[]  SumDenOutMin=[]  SumDenOutMax=[]  SumNumOutMin=[]  SumNumOutMax=[]  DivideOutMin=[]  DivideOutMax=[]  UdiffTsProdOutMin=[]  UdiffTsProdOutMax=[]  NTsProdOutMin=[]  NTsProdOutMax=[]  UintegralTsProdOutMin=[]  UintegralTsProdOutMax=[]  UngainTsProdOutMin=[]  UngainTsProdOutMax=[]  ClampingZeroOutDataTypeStr=Inherit: Inherit via back propagation  ClampingZeroOutMin=[]  ClampingZeroOutMax=[]  FilterDenConstantOutDataTypeStr=Inherit: Inherit via back propagation  FilterDenConstantOutMin=[]  FilterDenConstantOutMax=[]  PCopyOutDataTypeStr=Inherit: Inherit via back propagation  PCopyOutMin=[]  PCopyOutMax=[]  NCopyOutDataTypeStr=Inherit: Inherit via back propagation  NCopyOutMin=[]  NCopyOutMax=[]  IntegratorContinuousStateAttributes=''  IntegratorStateMustResolveToSignalObject=off  IntegratorRTWStateStorageClass=Auto  FilterContinuousStateAttributes=''  FilterStateMustResolveToSignalObject=off  FilterRTWStateStorageClass=Auto  ParallelPVariant=InternalParameters  IdealPVariant=Disabled  IVariant=InternalParameters  DVariant=Disabled  IntegratorVariant=Discrete  SatVariant=Enabled  AWVariant=DiscClampingParallel  PCopyVariant=Disabled  TRVariant=Disabled  FdbkBlocksVariant=Forward  IdealPFdbkVariant=Disabled  SatFdbkVariant=Disabled  DerivativeFilterVariant=Disabled  NVariant=Disabled  NCopyVariant=Disabled_SignalSpec  FilterICVariant=Disabled  IntegratorICVariant=InternalICs  ExternalResetVariant=Disabled  TRSumVariant=Passthrough  SumFdbkVariant=Disabled  SumVariant=Sum_PI  TsampFilterVariant=InternalTs  TsampNgainVariant=Passthrough  TsampIntegralVariant=Disabled_SignalSpec  ExternalSaturationOutDataTypeStr=Inherit: Same as second input  DerivativeSourceVariant=Disabled
  PWM Generator (DC-DC) : spsPWMGeneratorDCDCLib/PWM Generator (DC-DC)  Fsw=fs_mppt  Ts=0
  Product : Product
  Series RLC Branch1 : spsSeriesRLCBranchLib/Series RLC Branch  LConnTagsString=__new0  RConnTagsString=__new0  BranchType=L  Resistance=0.001  Inductance=L_mppt  SetiL0=off  InitialCurrent=0  Capacitance=50e-3  Setx0=off  InitialVoltage=0  Measurements=Branch current
  Series RLC Branch4 : spsSeriesRLCBranchLib/Series RLC Branch  LConnTagsString=__new0  RConnTagsString=__new0  BranchType=RC  Resistance=0.001  Inductance=1e-3  SetiL0=off  InitialCurrent=0  Capacitance=C_mppt  Setx0=off  InitialVoltage=900  Measurements=Branch voltage
  Series RLC Branch5 : spsSeriesRLCBranchLib/Series RLC Branch  LConnTagsString=__new0  RConnTagsString=__new0  BranchType=C  Resistance=0.001  Inductance=1e-3  SetiL0=off  InitialCurrent=0  Capacitance=C_mppt  Setx0=off  InitialVoltage=0  Measurements=None
  Unit Delay : UnitDelay  SampleTime=1e-5  HasFrameUpgradeWarning=on
  Unit Delay1 : UnitDelay  SampleTime=1e-5  HasFrameUpgradeWarning=on
  Voltage Measurement1 : spsVoltageMeasurementLib/Voltage Measurement  PhasorSimulation=off  OutputType=Complex  PSBequivalent=0
  PV : PMIOPort  Side=Left
  out : PMIOPort  Port=2  Side=Right
  tag scope: Ppv=global
  wires:
  PWM Generator (DC-DC)/1 -> IGBT/1
  Unit Delay1/1 -> MATLAB Function/2(Ipv)
  PID Controller/1 -> PWM Generator (DC-DC)/1
  Add/1 -> PID Controller/1
  Unit Delay/1 -> MATLAB Function/1(Vpv), Add/1
  MATLAB Function/1(Vref) -> Add/2
  Voltage Measurement1/1 -> Product/1, Unit Delay/1
  Current Measurement/1 -> Product/2, Unit Delay1/1
  Product/1 -> [Ppv]
  connections:
  Voltage Measurement1/LConn1 -- PV/RConn1 -- Current Measurement/LConn1
  Series RLC Branch4/RConn1 -- Ground8/LConn1
  Diode/LConn1 -- Series RLC Branch1/RConn1 -- IGBT/LConn1
  Series RLC Branch5/LConn1 -- out/RConn1 -- Diode/RConn1
  Series RLC Branch1/LConn1 -- Current Measurement/RConn1 -- Series RLC Branch4/LConn1
  Ground/LConn1 -- Voltage Measurement1/LConn2
  Series RLC Branch5/RConn1 -- Ground2/LConn1
  IGBT/RConn1 -- Ground1/LConn1

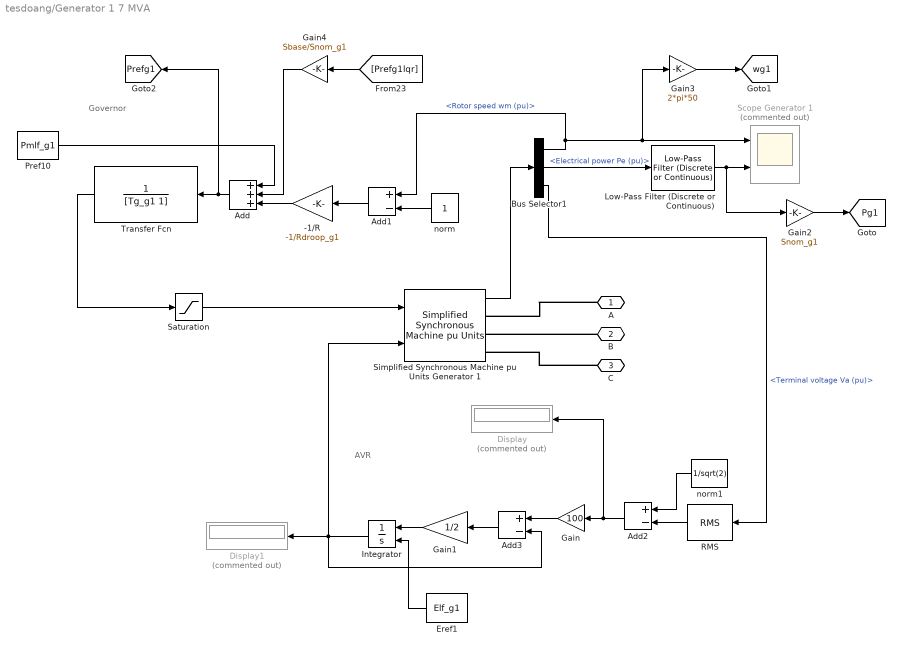
== system tesdoang/Generator 1 7 MVA ==
  note: AVR
  note: Governor
  -1/R : Gain  Gain=-1/Rdroop_g1
  Add : Sum  Inputs=+++
  Add1 : Sum  Inputs=+-
  Add2 : Sum  Inputs=+-
  Add3 : Sum  Inputs=+-
  Bus Selector1 : BusSelector  OutputSignals=Rotor speed wm (pu),Electrical power Pe (pu),Terminal voltage Va (pu)
  Display : Display  Commented=on
  Display1 : Display  Commented=on
  Eref1 : Constant  Value=Elf_g1  SampleTime=1e-6
  Gain : Gain  Gain=100
  Gain1 : Gain  Gain=1/2
  Gain2 : Gain  Gain=Snom_g1
  Gain3 : Gain  Gain=2*pi*50
  Gain4 : Gain  Gain=Sbase/Snom_g1
  Integrator : Integrator  InitialConditionSource=external  InitialCondition=Elf_g1  LimitOutput=on  UpperSaturationLimit=1.3  LowerSaturationLimit=0.7
  Low-Pass Filter (Discrete or Continuous) : eeGeneralControl/Low-Pass Filter (Discrete or Continuous)  K=1  T=1/(2*pi*15)  B=inf  A=-inf  init_option=Inherited from block input  x0=0  Ts=-1
  Pref10 : Constant  Value=Pmlf_g1  SampleTime=1e-6
  RMS : spsRMSLib/RMS  TrueRMS=on  Freq=50  RMSInit=0.707  Ts=1e-6
  Saturation : Saturate  UpperLimit=1.1  LowerLimit=0.05
  Scope Generator 1 : Scope  Commented=on  NumInputPorts=2
  Simplified Synchronous Machine pu Units Generator 1 : spsSimplifiedSynchronousMachinepuUnitsLib/Simplified Synchronous Machine pu Units  ConnectionType=3-wire Y  MechanicalLoad=Mechanical power Pm  MeasurementBus=off  NominalParameters=[Snom_g1 Vac_grid fg]  Mechanical=[H_g1 D_g1 pairPoles_g1]  InternalRL="[R_g1  X_g1]"  InitialConditions=[0 13.769 0.815534 0.815534 0.815534 2.94225 -117.058 122.942]  IterativeDiscreteModel=Trapezoidal non iterative  TsBlock=1e-6  TsPowergui=0  LoadFlowParameters=[1,0,0,0,0]  Units=0  BusType=swing  Pref=6000000  Qref=0  Qmin=-2100000  Qmax=2800000  PLF=0  QLF=0
      settings: LibrarySourceBlock=|
      | sps_lib/Electrical Machines/Simplified Synchronous
      | Machine pu Units
  Transfer Fcn : TransferFcn  Denominator=[Tg_g1 1]
  norm : Constant  SampleTime=1e-6
  norm1 : Constant  Value=1/sqrt(2)  SampleTime=1e-6
  A : PMIOPort  Side=Right
  B : PMIOPort  Port=2  Side=Right
  C : PMIOPort  Port=3  Side=Right
  tag scope: Pg1=global, Prefg1=global, wg1=global
  wires:
  Transfer Fcn/1 -> Saturation/1
  Bus Selector1/1 -> Add1/1, Gain3/1, Scope Generator 1/1  "<Rotor speed wm (pu)>"
  Bus Selector1/2 -> Low-Pass Filter (Discrete or Continuous)/1  "<Electrical power Pe (pu)>"
  Simplified Synchronous Machine pu Units Generator 1/1 -> Bus Selector1/1
  Add/1 -> [Prefg1], Transfer Fcn/1
  -1/R/1 -> Add/3
  norm/1 -> Add1/2
  Add1/1 -> -1/R/1
  Saturation/1 -> Simplified Synchronous Machine pu Units Generator 1/1
  Pref10/1 -> Add/1
  Low-Pass Filter (Discrete or Continuous)/1 -> Gain2/1, Scope Generator 1/2
  Bus Selector1/3 -> RMS/1  "<Terminal voltage Va (pu)>"
  RMS/1 -> Add2/2
  norm1/1 -> Add2/1
  Add2/1 -> Display/1, Gain/1
  Gain/1 -> Add3/1
  Add3/1 -> Gain1/1
  Gain1/1 -> Integrator/1
  Integrator/1 -> Simplified Synchronous Machine pu Units Generator 1/2, Display1/1, Add3/2
  Eref1/1 -> Integrator/2
  Gain2/1 -> [Pg1]
  Gain3/1 -> [wg1]
  [Prefg1lqr] -> Gain4/1
  Gain4/1 -> Add/2
  connections:
  A/RConn1 -- Simplified Synchronous Machine pu Units Generator 1/RConn1
  C/RConn1 -- Simplified Synchronous Machine pu Units Generator 1/RConn3
  B/RConn1 -- Simplified Synchronous Machine pu Units Generator 1/RConn2

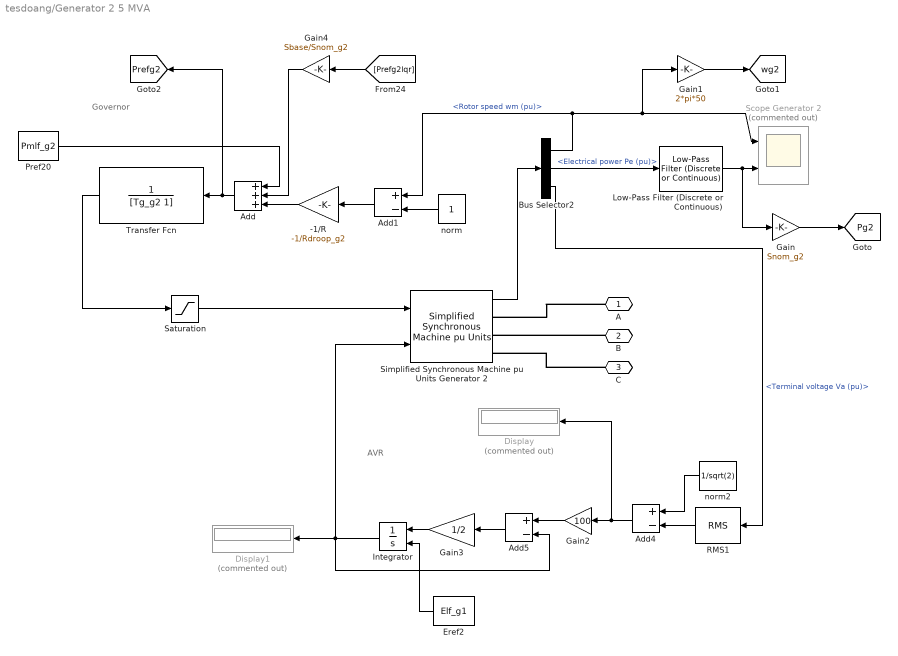
== system tesdoang/Generator 2 5 MVA ==
  note: AVR
  note: Governor
  -1/R : Gain  Gain=-1/Rdroop_g2
  Add : Sum  Inputs=+++
  Add1 : Sum  Inputs=+-
  Add4 : Sum  Inputs=+-
  Add5 : Sum  Inputs=+-
  Bus Selector2 : BusSelector  OutputSignals=Rotor speed wm (pu),Electrical power Pe (pu),Terminal voltage Va (pu)
  Display : Display  Commented=on
  Display1 : Display  Commented=on
  Eref2 : Constant  Value=Elf_g1  SampleTime=1e-6
  Gain : Gain  Gain=Snom_g2
  Gain1 : Gain  Gain=2*pi*50
  Gain2 : Gain  Gain=100
  Gain3 : Gain  Gain=1/2
  Gain4 : Gain  Gain=Sbase/Snom_g2
  Integrator : Integrator  InitialConditionSource=external  InitialCondition=Elf_g2  LimitOutput=on  UpperSaturationLimit=1.3  LowerSaturationLimit=0.7
  Low-Pass Filter (Discrete or Continuous) : eeGeneralControl/Low-Pass Filter (Discrete or Continuous)  K=1  T=1/(2*pi*15)  B=inf  A=-inf  init_option=Inherited from block input  x0=0  Ts=-1
  Pref20 : Constant  Value=Pmlf_g2  SampleTime=1e-6
  RMS1 : spsRMSLib/RMS  TrueRMS=on  Freq=50  RMSInit=0.707  Ts=1e-6
  Saturation : Saturate  UpperLimit=1.1  LowerLimit=0.05
  Scope Generator 2 : Scope  Commented=on  NumInputPorts=2
  Simplified Synchronous Machine pu Units Generator 2 : spsSimplifiedSynchronousMachinepuUnitsLib/Simplified Synchronous Machine pu Units  ConnectionType=3-wire Y  MechanicalLoad=Mechanical power Pm  MeasurementBus=off  NominalParameters=[Snom_g2 Vac_grid fg]  Mechanical=[H_g2 D_g2 pairPoles_g2]  InternalRL="[R_g2  X_g2]"  InitialConditions=[0 13.9078 0.837652 0.837652 0.837652 -17.3386 -137.339 102.661]  IterativeDiscreteModel=Trapezoidal non iterative  TsBlock=1e-6  TsPowergui=0  LoadFlowParameters=[1,0,0,0,0]  Units=0  BusType=PV  Pref=4000000  Qref=0  Qmin=-1250000  Qmax=1500000  PLF=0  QLF=0
      settings: LibrarySourceBlock=|
      | sps_lib/Electrical Machines/Simplified Synchronous
      | Machine pu Units
  Transfer Fcn : TransferFcn  Denominator=[Tg_g2 1]
  norm : Constant  SampleTime=1e-6
  norm2 : Constant  Value=1/sqrt(2)  SampleTime=1e-6
  A : PMIOPort  Side=Right
  B : PMIOPort  Port=2  Side=Right
  C : PMIOPort  Port=3  Side=Right
  tag scope: Pg2=global, Prefg2=global, wg2=global
  wires:
  Bus Selector2/1 -> Add1/1, Gain1/1, Scope Generator 2/1  "<Rotor speed wm (pu)>"
  Simplified Synchronous Machine pu Units Generator 2/1 -> Bus Selector2/1
  norm/1 -> Add1/2
  Add1/1 -> -1/R/1
  Add/1 -> [Prefg2], Transfer Fcn/1
  -1/R/1 -> Add/3
  Bus Selector2/2 -> Low-Pass Filter (Discrete or Continuous)/1  "<Electrical power Pe (pu)>"
  Transfer Fcn/1 -> Saturation/1
  Saturation/1 -> Simplified Synchronous Machine pu Units Generator 2/1
  Pref20/1 -> Add/1
  Bus Selector2/3 -> RMS1/1  "<Terminal voltage Va (pu)>"
  norm2/1 -> Add4/1
  RMS1/1 -> Add4/2
  Add4/1 -> Display/1, Gain2/1
  Gain3/1 -> Integrator/1
  Integrator/1 -> Simplified Synchronous Machine pu Units Generator 2/2, Display1/1, Add5/2
  Gain2/1 -> Add5/1
  Add5/1 -> Gain3/1
  Eref2/1 -> Integrator/2
  Low-Pass Filter (Discrete or Continuous)/1 -> Gain/1, Scope Generator 2/2
  Gain/1 -> [Pg2]
  Gain1/1 -> [wg2]
  [Prefg2lqr] -> Gain4/1
  Gain4/1 -> Add/2
  connections:
  B/RConn1 -- Simplified Synchronous Machine pu Units Generator 2/RConn2
  A/RConn1 -- Simplified Synchronous Machine pu Units Generator 2/RConn1
  C/RConn1 -- Simplified Synchronous Machine pu Units Generator 2/RConn3
